simulink model "LinearWhiteNoise"  (R2015b)
settings: Solver=VariableStepAuto  StartTime=0.0  StopTime=10.0  RelTol=1e-3
settings Model: Creator=HP  LastModifiedBy=HP

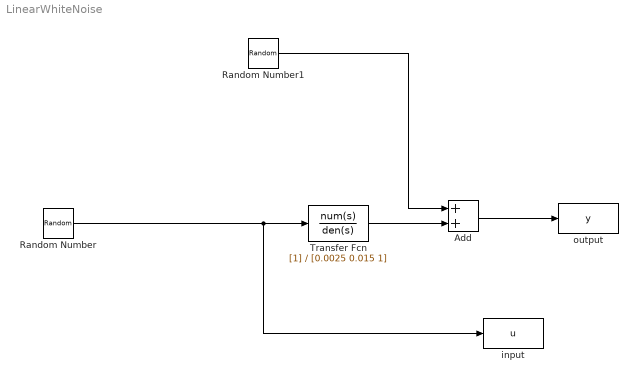
== system LinearWhiteNoise ==
  Add : Sum
  Random Number : RandomNumber  SampleTime=0.01
  Random Number1 : RandomNumber  Variance=0.01  Seed=1  SampleTime=0.01
  Transfer Fcn : TransferFcn  Denominator=[0.0025 0.015 1]
  input : ToWorkspace  VariableName=u  SaveFormat=Timeseries  SampleTime=-1
  output : ToWorkspace  VariableName=y  SaveFormat=Timeseries  SampleTime=-1
  wires:
  Random Number/1 -> input/1, Transfer Fcn/1
  Transfer Fcn/1 -> Add/2
  Random Number1/1 -> Add/1
  Add/1 -> output/1
